simulink library "coordinate_transforms"  (R2021b)
settings: Solver=VariableStepAuto  StartTime=0.0  StopTime=10.0  RelTol=1e-3
settings Model: Creator=Nikita  LastModifiedBy=Nikita
settings SolverCC: AlgebraicLoopSolver=TrustRegion
settings DebuggingCC: SFMachineParentedDataDiag=warning

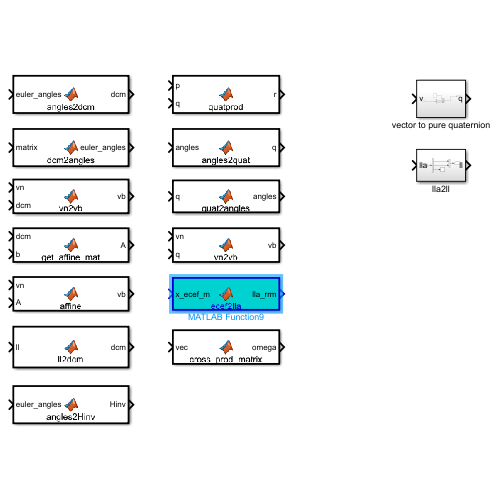
[thumbnail: Simulink's stored preview of the top-level diagram]
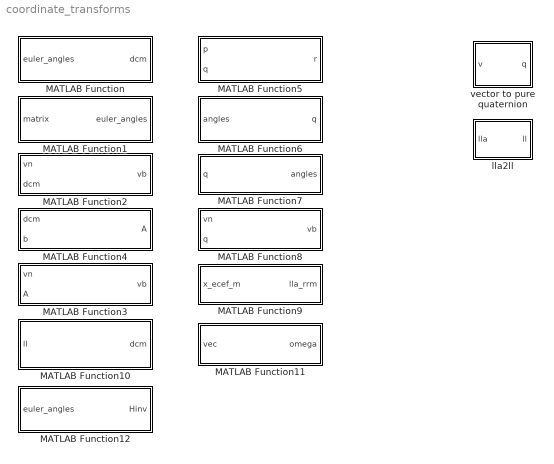
== system coordinate_transforms ==
  MATLAB Function : MATLAB Function  TreatAsAtomicUnit=on
  MATLAB Function1 : MATLAB Function  TreatAsAtomicUnit=on
  MATLAB Function10 : MATLAB Function  TreatAsAtomicUnit=on
  MATLAB Function11 : MATLAB Function  TreatAsAtomicUnit=on
  MATLAB Function12 : MATLAB Function  TreatAsAtomicUnit=on
  MATLAB Function2 : MATLAB Function  TreatAsAtomicUnit=on
  MATLAB Function3 : MATLAB Function  TreatAsAtomicUnit=on
  MATLAB Function4 : MATLAB Function  TreatAsAtomicUnit=on
  MATLAB Function5 : MATLAB Function  TreatAsAtomicUnit=on
  MATLAB Function6 : MATLAB Function  TreatAsAtomicUnit=on
  MATLAB Function7 : MATLAB Function  TreatAsAtomicUnit=on
  MATLAB Function8 : MATLAB Function  TreatAsAtomicUnit=on
  MATLAB Function9 : MATLAB Function  TreatAsAtomicUnit=on
  lla2ll : Subsystem
  vector to pure quaternion : Subsystem

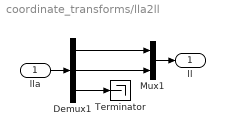
== system coordinate_transforms/lla2ll ==
  lla : Inport
  Demux1 : Demux  Outputs=3
  Mux1 : Mux  Inputs=2
  Terminator : Terminator
  ll : Outport
  wires:
  Demux1/1 -> Mux1/1
  Mux1/1 -> ll/1
  Demux1/3 -> Terminator/1
  Demux1/2 -> Mux1/2
  lla/1 -> Demux1/1

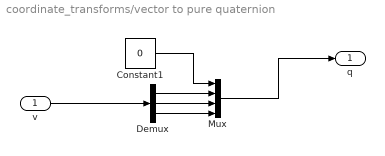
== system coordinate_transforms/vector to pure quaternion ==
  v : Inport
  Constant1 : Constant  Value=0
  Demux : Demux  Outputs=3
  Mux : Mux
  q : Outport
  wires:
  Demux/2 -> Mux/3
  Demux/1 -> Mux/2
  Constant1/1 -> Mux/1
  Demux/3 -> Mux/4
  v/1 -> Demux/1
  Mux/1 -> q/1

== matlab function coordinate_transforms/MATLAB Function ==
  data: euler_angles input; dcm output
% Enter the euler_angles as follows: yaw; pitch; roll
function dcm = angles2dcm(euler_angles)
yaw     = euler_angles(1);
pitch   = euler_angles(2);
roll    = euler_angles(3);

roll_matrix     = [1, 0, 0; 
                0, cos(roll), sin(roll); 
                0, -sin(roll), cos(roll)];
            
pitch_matrix    = [cos(pitch), 0, -sin(pitch); 
                0, 1, 0; 
                sin(pitch), 0, cos(pitch)];
            
yaw_matrix      = [cos(yaw), sin(yaw), 0; 
                -sin(yaw), cos(yaw), 0; 
                0, 0, 1];

% yaw-pitch-roll sequence
dcm = roll_matrix*pitch_matrix*yaw_matrix;

== matlab function coordinate_transforms/MATLAB Function2 ==
  data: vn input; vb output; dcm input
% change vector v in N frame to a vector in the B frame usingn a DCM from
% the N frame to the B frame
function vb = vn2vb(vn, dcm)

vb = dcm*vn;

== matlab function coordinate_transforms/MATLAB Function3 ==
  data: vn input; vb output; A input
% complete an affine transformation
%
% vn: original vector
% A: affine transformation matrix
%
% vb: vector after affine transformation
function vb = affine(vn, A)

vb = A*vn;

== matlab function coordinate_transforms/MATLAB Function4 ==
  data: dcm input; A output; b input
% Get the affine transformation matrix A from the rotation dcm and
% translation vector b
function A = get_affine_mat(dcm, b)

A = [dcm, b; 0, 0, 0, 1];

== matlab function coordinate_transforms/MATLAB Function5 ==
  data: p input; r output; q input
%% Quaternion multiplication
% Equivalent to coordinate transforms with quaternions
% p must be a vector of length 4
% q must be a column vector of length 4
function r = quatprod(p, q)

p_matrix = [p(1), -p(2), -p(3), -p(4);
            p(2),  p(1), -p(4),  p(3);
            p(3),  p(4),  p(1), -p(2);
            p(4), -p(3),  p(2),  p(1)];

r = p_matrix*q; % Formula just before 1.8-3b in the book

== matlab function coordinate_transforms/MATLAB Function6 ==
  data: angles input; q output
% Get quaternion from Euler angles.
% Angles must be in this order: yaw, pitch, roll.
function q = angles2quat(angles)
yaw     = angles(1); % psi
pitch   = angles(2); % theta
roll    = angles(3); % phi

q = [cos(roll/2)*cos(pitch/2)*cos(yaw/2) ...
    + sin(roll/2)*sin(pitch/2)*sin(yaw/2);
    
    sin(roll/2)*cos(pitch/2)*cos(yaw/2) ...
    - cos(roll/2)*sin(pitch/2)*sin(yaw/2);
    
    cos(roll/2)*sin(pitch/2)*cos(yaw/2) ...
    + sin(roll/2)*cos(pitch/2)*sin(yaw/2);
    
    cos(roll/2)*cos(pitch/2)*sin(yaw/2) ...
    - sin(roll/2)*sin(pitch/2)*cos(yaw/2);
    ];

== matlab function coordinate_transforms/MATLAB Function7 ==
  data: q input; angles output
function angles = quat2angles(q)

c_23 = 2*(q(3)*q(4) + q(1)*q(2)); % was -
c_33 = (q(1)^2 - q(2)^2 - q(3)^2 + q(4)^2);

c_13 = 2*(q(2)*q(4) - q(1)*q(3));
c_12 = 2*(q(2)*q(3) + q(1)*q(4));
c_11 = (q(1)^2 + q(2)^2 - q(3)^2 - q(4)^2);

phi     = atan2(c_23, c_33);
theta   = -asin(c_13);
psi     = atan2(c_12, c_11);

angles = [psi; theta; phi];

== matlab function coordinate_transforms/MATLAB Function8 ==
  data: vn input; vb output; q input
function vb = vn2vb(vn, q)

    q_inv   = [q(1); -q(2); -q(3); -q(4)];
    vn_e    = [0;    vn(1); vn(2); vn(3)];

    vb = quatprod(quatprod(q_inv,vn_e), q);
end

function r = quatprod(p, q)
    p_matrix = [p(1), -p(2), -p(3), -p(4);
                p(2),  p(1), -p(4),  p(3);
                p(3),  p(4),  p(1), -p(2);
                p(4), -p(3),  p(2),  p(1)];

    r = p_matrix*q; % Formula just before 1.8-3b in the book
end

== matlab function coordinate_transforms/MATLAB Function9 ==
  data: x_ecef_m input; lla_rrm output
% Custom MATLAB function to convert from rectangular coordinates in ecef to
% latitude longitude altitude (lla) in degrees, degrees, meters
function lla_rrm = ecef2lla(x_ecef_m)

re_m = 6378000; %TODO implement constants

r = norm(x_ecef_m);
lat = asin(x_ecef_m(3)/r)*180/pi;
lon = atan2(x_ecef_m(2), x_ecef_m(1))*180/pi;
r = norm(x_ecef_m) - re_m;

lla_rrm = [lat; lon; r];

== matlab function coordinate_transforms/MATLAB Function1 ==
  data: matrix input; euler_angles output
% output is yaw pitch roll (psi theta phi)
function euler_angles = dcm2angles(matrix)
phi     = atan2(matrix(2,3), matrix(3,3));
theta   = -asin(matrix(1,3));
psi     = atan2(matrix(1,2), matrix(1,1));

euler_angles = [psi; theta; phi]; % yaw pitch roll

== matlab function coordinate_transforms/MATLAB Function10 ==
  data: ll input; dcm output
% Enter the latitude ang longitude for a DCM from ECEF to NED
function dcm = ll2dcm(ll)

% Yaw (about ECEF Z) starts at 0 degrees about Z, and is positive longitude
yaw     = ll(2)*pi/180; 
% Pitch (about ECEF Y) starts at -90 degrees about Y, and latitude is 
% negative pitch 
pitch   = -pi/2-ll(1)*pi/180; 
% Roll (about ECEF X) stays 0
roll    = 0; 

roll_matrix     = [1, 0, 0; 
                0, cos(roll), sin(roll); 
                0, -sin(roll), cos(roll)];
            
pitch_matrix    = [cos(pitch), 0, -sin(pitch); 
                0, 1, 0; 
                sin(pitch), 0, cos(pitch)];
            
yaw_matrix      = [cos(yaw), sin(yaw), 0; 
                -sin(yaw), cos(yaw), 0; 
                0, 0, 1];

% yaw-pitch-roll sequence
dcm = roll_matrix*pitch_matrix*yaw_matrix;

== matlab function coordinate_transforms/MATLAB Function11 ==
  data: vec input; omega output
function omega = cross_prod_matrix(vec)

omega = [0,     -vec(3), vec(2);
         vec(3), 0,     -vec(1);
        -vec(2), vec(1), 0];

== matlab function coordinate_transforms/MATLAB Function12 ==
  data: euler_angles input; Hinv output
%euler angles must be in yaw pitch roll order
function Hinv = angles2Hinv(euler_angles)

psi     = euler_angles(1);
theta   = euler_angles(2);
phi     = euler_angles(3);

Hinv = [1, tan(theta)*sin(phi), tan(theta)*cos(phi);
        0, cos(phi),            -sin(phi);
        0, sin(phi)/cos(theta), cos(phi)/cos(theta)];
